simulink model "hybrid_ac_dc_microgrid"  (R2017b)
settings: Solver=ode4  StartTime=0.0  StopTime=4  RelTol=1e-3
model workspace (MAT data in the model file):
  Ts = 1e-06
undefined symbols (not defined in the file or in its folder): Acid, Clink, D1, Delta, DiscIntNeverNeededParam, find_system, Lead, Vnom_dc
libraries: powerlib x42, powerlib_extras x36, powerlib_meascontrol x14, simulink x8, simulink_extras x6, electricdrivelib x1, re_lib x1
(part 4 of 4)

== matlab function hybrid_ac_dc_microgrid/Double stage Grid connected Solar PV Array with Bateery /Inverter Control/MPPT Controller using Perturbe & Observe technique  ==
  settings: updateMethod=DISCRETE  sampleTime=Ts_Control
  data: Param input; Enabled input; V input =V; I input; D output
function D  = PandO(Param, Enabled, V, I)

% MPPT controller based on the Perturb & Observe algorithm.

% D output = Reference for DC link voltage (Vdc_ref) 
%
% Enabled input = 1 to enable the MPPT controller
% V input = PV array terminal voltage (V)
% I input = PV array current (A)
%
% Param input:
Dinit = Param(1);  %Initial value for Vdc_ref
Dmax = Param(2);   %Maximum value for Vdc_ref
Dmin = Param(3);   %Minimum value for Vdc_ref
deltaD = Param(4); %Increment value used to increase/decrease Vdc_ref
%  

persistent Vold Pold Dold;

dataType = 'double';

if isempty(Vold)
    Vold=0;
    Pold=0;
    Dold=Dinit;
end
P= V*I;
dV= V - Vold;
dP= P - Pold;

if dP ~= 0 & Enabled ~=0
    if dP < 0
        if dV < 0
            D = Dold + deltaD;
        else
            D = Dold - deltaD;
        end
    else
        if dV < 0
            D = Dold - deltaD;
        else
            D = Dold + deltaD;
        end    
    end
else D=Dold;
end

if D >= Dmax | D<= Dmin
    D=Dold;
end

Dold=D;
Vold=V;
Pold=P;

== stateflow chart hybrid_ac_dc_microgrid/Double stage Grid connected Solar PV Array with Bateery /Inverter Control/Chart ==
  state Fromgrid
    entry:
    Idref=-0.5
  state Togrid
    entry:
    Idref=0.5
  (default) -> Fromgrid
  Fromgrid -> Togrid : [SOC>70]
  Togrid -> Fromgrid : [SOC<30]
  data: Idref output; SOC input
